simulink model "master"  (R2020a)
settings: Solver=FixedStepDiscrete  StartTime=0.0  StopTime=10.0  FixedStep=1000  MaxStep=0.2  RelTol=1e-3  EnableMultiTasking=on
settings Model: SILPILModeSetting=veronly  ExtModeTrigDuration=2  Creator=Yalda  LastModifiedBy=Yalda
settings OptimizationCC: DefaultParameterBehavior=Inlined  UseDivisionForNetSlopeComputation=on  GainParamInheritBuiltInType=on  UseFloatMulNetSlope=on  InlineInvariantSignals=on  PassReuseOutputArgsAs=Individual arguments  ZeroExternalMemoryAtStartup=off  ZeroInternalMemoryAtStartup=off  NoFixptDivByZeroProtection=on  EfficientFloat2IntCast=on  LifeSpan=1  MaxStackSize=64  OptimizeBlockOrder=speed  DifferentSizesBufferReuse=on  EfficientTunableParamExpr=on
settings DebuggingCC: ParameterTunabilityLossMsg=error
settings HardwareCC: ProdBitPerInt=16  ProdBitPerPointer=16  ProdBitPerSizeT=16  ProdBitPerPtrDiffT=16  ProdLargestAtomicFloat=None  ProdWordSize=8  ProdLongLongMode=on  ProdHWDeviceType=Atmel->AVR
settings SFSimCC: MATLABDynamicMemAlloc=off
settings RTWCC: SystemTargetFile=ert.tlc  HardwareBoard=Arduino Uno  TLCOptions=-aInlineSetEventsForThisBaseRateFcn=TLC_FALSE -aSuppressMultiTaskScheduler=TLC_FALSE -aRateBasedStepFcn=1  TemplateMakefile=ert_default_tmf  Toolchain=Arduino AVR  BuildConfiguration=Faster Runs
settings CodeAppCC: ForceParamTrailComments=on  IgnoreCustomStorageClasses=off  OperatorAnnotations=on  SimulinkDataObjDesc=on  SFDataObjDesc=on  CustomSymbolStrGlobalVar=rt$N$M  CustomSymbolStrType=$N$M  CustomSymbolStrFcn=$N$M$F  CustomSymbolStrMacro=$N$M  InsertBlockDesc=on
settings ERTTargetCC: IncludeMdlTerminateFcn=off  CombineSignalStateStructs=on  SupportAbsoluteTime=off  PurelyIntegerCode=on  SupportComplex=off  SupportNonInlinedSFcns=on  ExtModeStaticAllocSize=250  InlinedParameterPlacement=NonHierarchical  ERTFilePackagingFormat=CompactWithDataFile

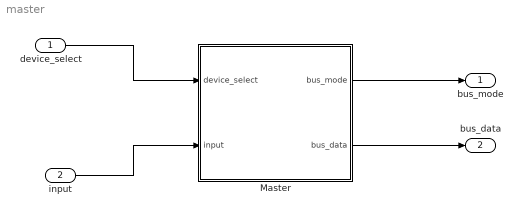
== system master ==
  device_select : Inport
  input : Inport  Port=2
  Master : Subsystem
  bus_mode : Outport
  bus_data : Outport  Port=2
  wires:
  device_select/1 -> Master/1(device_select)
  input/1 -> Master/2(input)
  Master/1(bus_mode) -> bus_mode/1
  Master/2(bus_data) -> bus_data/1

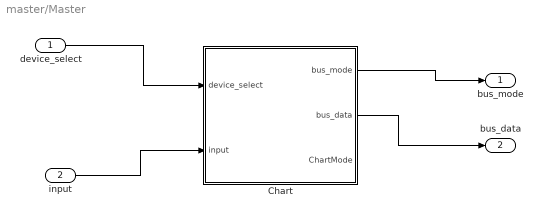
== system master/Master ==
  device_select : Inport
  input : Inport  Port=2
  Chart : Stateflow chart  TreatAsAtomicUnit=on
  bus_mode : Outport
  bus_data : Outport  Port=2
  wires:
  Chart/1(bus_mode) -> bus_mode/1
  input/1 -> Chart/2(input)
  device_select/1 -> Chart/1(device_select)
  Chart/2(bus_data) -> bus_data/1

== stateflow chart master/Master/Chart ==
  state free
  state startSending
  state sendCommand
  state monitor
  state sendAddr
  (default) -> free : {bus_mode=1;}
  free -> startSending : [device_select==1 || device_select==2]{bus_data=1;}
  sendCommand -> free [order 2] : [device_select == 1 || device_select == 2]{bus_data=0}
  startSending -> sendAddr : {bus_data=address;}
  monitor -> sendCommand : {bus_mode=1; bus_data=input}
  sendAddr -> monitor : {bus_mode=0;}
  sendCommand -> monitor [order 1] : [device_select != 1 && device_select != 2]{bus_mode=0}
  data: address local uint8; device_select input uint8; input input uint8; bus_mode output uint8; bus_data output uint8; ChartMode output Enum: ChartModeType
